simulink model "simRouteA_v4_11"  (R2015a)
settings: Solver=FixedStepDiscrete  StartTime=0.0  StopTime=36000  FixedStep=1  RelTol=1e-3
PreLoadFcn:
  | loadTimetable
StopFcn:
  | postProcess
undefined symbols (not defined in the file or in its folder): setBus1IntergenTime, setBus2IntergenTime, setBus3IntergenTime, setBus4IntergenTime
(part 3 of 7)

== system simRouteA_v4_11/inTransitLinkL10 ==
  xtraDelay : Inport
  theoTravTime : Inport  Port=2
  Add : Sum
  Buses being hold on the street : InfiniteServer  ServiceTimeFrom=Signal port t
  Clock2 : Clock
  DummyServer : SingleServer  ServiceTime=0
  FIFO Queue1 : FIFOQueue
  FIFO Queue3 : FIFOQueue
  FIFO Queue9 : FIFOQueue
  Get Attribute : GetAttribute  AttributeName=ID  EvaluatedDefaultAttributeValue={ []}
      settings: OutputPortMap=o1
  Get Attribute5 : GetAttribute  AttributeName=tTrav|time  AttributeMissing=Error|Error  AttributeDefaultValue=1|1  AttributeTreatAsVector=1|1  AttributeSendTiming=After entity departure|After entity departure  EvaluatedDefaultAttributeValue={ []; []}
      settings: OutputPortMap=o1,o2
  Set Attribute3 : SetAttribute  AttributeName=tTrav|time  AttributeFrom=Signal port|Signal port  AttributeValue=1|1  AttributeTreatAsVector=1|1  EvaluatedAttributeValue={ []; [] }
      settings: InputPortMap=u0,u1
  Subsystem2 : Subsystem  TreatAsAtomicUnit=on
  T2E4 : TimedToEventSignal
  busesOutLink : PMIOPort  Port=1  Side=Right
  busesHitTheRoad : PMIOPort  Port=2  Side=Left
  idBusOutLink : Outport
  wires:
  xtraDelay/1 -> Add/1
  theoTravTime/1 -> Add/2
  Add/1 -> Set Attribute3/1
  Get Attribute/1 -> idBusOutLink/1
  Clock2/1 -> T2E4/1
  T2E4/1 -> Set Attribute3/2
  Get Attribute5/1 -> Subsystem2/1(tTrav)
  Get Attribute5/2 -> Subsystem2/2(tDep)
  Subsystem2/1(tTravNew) -> Buses being hold on the street/1
  connections:
  Buses being hold on the street/RConn1 -- FIFO Queue9/LConn1
  FIFO Queue1/LConn1 -- busesHitTheRoad/RConn1
  Get Attribute/RConn1 -- busesOutLink/RConn1
  FIFO Queue9/RConn1 -- Get Attribute/LConn1
  FIFO Queue1/RConn1 -- Set Attribute3/LConn1
  Set Attribute3/RConn1 -- FIFO Queue3/LConn1
  FIFO Queue3/RConn1 -- Get Attribute5/LConn1
  Get Attribute5/RConn1 -- DummyServer/LConn1
  DummyServer/RConn1 -- Buses being hold on the street/LConn1

== system simRouteA_v4_11/inTransitLinkL11 ==
  xtraDelay : Inport
  theoTravTime : Inport  Port=2
  Add : Sum
  Buses being hold on the street : InfiniteServer  ServiceTimeFrom=Signal port t
  Clock2 : Clock
  DummyServer : SingleServer  ServiceTime=0
  FIFO Queue1 : FIFOQueue
  FIFO Queue3 : FIFOQueue
  FIFO Queue9 : FIFOQueue
  Get Attribute : GetAttribute  AttributeName=ID  EvaluatedDefaultAttributeValue={ []}
      settings: OutputPortMap=o1
  Get Attribute5 : GetAttribute  AttributeName=tTrav|time  AttributeMissing=Error|Error  AttributeDefaultValue=1|1  AttributeTreatAsVector=1|1  AttributeSendTiming=After entity departure|After entity departure  EvaluatedDefaultAttributeValue={ []; []}
      settings: OutputPortMap=o1,o2
  Set Attribute3 : SetAttribute  AttributeName=tTrav|time  AttributeFrom=Signal port|Signal port  AttributeValue=1|1  AttributeTreatAsVector=1|1  EvaluatedAttributeValue={ []; [] }
      settings: InputPortMap=u0,u1
  Subsystem2 : Subsystem  TreatAsAtomicUnit=on
  T2E4 : TimedToEventSignal
  busesOutLink : PMIOPort  Port=1  Side=Right
  busesHitTheRoad : PMIOPort  Port=2  Side=Left
  idBusOutLink : Outport
  wires:
  xtraDelay/1 -> Add/1
  theoTravTime/1 -> Add/2
  Add/1 -> Set Attribute3/1
  Get Attribute/1 -> idBusOutLink/1
  Clock2/1 -> T2E4/1
  T2E4/1 -> Set Attribute3/2
  Get Attribute5/1 -> Subsystem2/1(tTrav)
  Get Attribute5/2 -> Subsystem2/2(tDep)
  Subsystem2/1(tTravNew) -> Buses being hold on the street/1
  connections:
  Buses being hold on the street/RConn1 -- FIFO Queue9/LConn1
  FIFO Queue1/LConn1 -- busesHitTheRoad/RConn1
  Get Attribute/RConn1 -- busesOutLink/RConn1
  FIFO Queue9/RConn1 -- Get Attribute/LConn1
  FIFO Queue1/RConn1 -- Set Attribute3/LConn1
  Set Attribute3/RConn1 -- FIFO Queue3/LConn1
  FIFO Queue3/RConn1 -- Get Attribute5/LConn1
  Get Attribute5/RConn1 -- DummyServer/LConn1
  DummyServer/RConn1 -- Buses being hold on the street/LConn1

== system simRouteA_v4_11/inTransitLinkL12 ==
  xtraDelay : Inport
  theoTravTime : Inport  Port=2
  Add : Sum
  Buses being hold on the street : InfiniteServer  ServiceTimeFrom=Signal port t
  Clock2 : Clock
  DummyServer : SingleServer  ServiceTime=0
  FIFO Queue1 : FIFOQueue
  FIFO Queue3 : FIFOQueue
  FIFO Queue9 : FIFOQueue
  Get Attribute : GetAttribute  AttributeName=ID  EvaluatedDefaultAttributeValue={ []}
      settings: OutputPortMap=o1
  Get Attribute5 : GetAttribute  AttributeName=tTrav|time  AttributeMissing=Error|Error  AttributeDefaultValue=1|1  AttributeTreatAsVector=1|1  AttributeSendTiming=After entity departure|After entity departure  EvaluatedDefaultAttributeValue={ []; []}
      settings: OutputPortMap=o1,o2
  Set Attribute3 : SetAttribute  AttributeName=tTrav|time  AttributeFrom=Signal port|Signal port  AttributeValue=1|1  AttributeTreatAsVector=1|1  EvaluatedAttributeValue={ []; [] }
      settings: InputPortMap=u0,u1
  Subsystem2 : Subsystem  TreatAsAtomicUnit=on
  T2E4 : TimedToEventSignal
  busesOutLink : PMIOPort  Port=1  Side=Right
  busesHitTheRoad : PMIOPort  Port=2  Side=Left
  idBusOutLink : Outport
  wires:
  xtraDelay/1 -> Add/1
  theoTravTime/1 -> Add/2
  Add/1 -> Set Attribute3/1
  Get Attribute/1 -> idBusOutLink/1
  Clock2/1 -> T2E4/1
  T2E4/1 -> Set Attribute3/2
  Get Attribute5/1 -> Subsystem2/1(tTrav)
  Get Attribute5/2 -> Subsystem2/2(tDep)
  Subsystem2/1(tTravNew) -> Buses being hold on the street/1
  connections:
  Buses being hold on the street/RConn1 -- FIFO Queue9/LConn1
  FIFO Queue1/LConn1 -- busesHitTheRoad/RConn1
  Get Attribute/RConn1 -- busesOutLink/RConn1
  FIFO Queue9/RConn1 -- Get Attribute/LConn1
  FIFO Queue1/RConn1 -- Set Attribute3/LConn1
  Set Attribute3/RConn1 -- FIFO Queue3/LConn1
  FIFO Queue3/RConn1 -- Get Attribute5/LConn1
  Get Attribute5/RConn1 -- DummyServer/LConn1
  DummyServer/RConn1 -- Buses being hold on the street/LConn1

== system simRouteA_v4_11/inTransitLinkL13 ==
  xtraDelay : Inport
  theoTravTime : Inport  Port=2
  Add : Sum
  Buses being hold on the street : InfiniteServer  ServiceTimeFrom=Signal port t
  Clock2 : Clock
  DummyServer : SingleServer  ServiceTime=0
  FIFO Queue1 : FIFOQueue
  FIFO Queue3 : FIFOQueue
  FIFO Queue9 : FIFOQueue
  Get Attribute : GetAttribute  AttributeName=ID  EvaluatedDefaultAttributeValue={ []}
      settings: OutputPortMap=o1
  Get Attribute5 : GetAttribute  AttributeName=tTrav|time  AttributeMissing=Error|Error  AttributeDefaultValue=1|1  AttributeTreatAsVector=1|1  AttributeSendTiming=After entity departure|After entity departure  EvaluatedDefaultAttributeValue={ []; []}
      settings: OutputPortMap=o1,o2
  Set Attribute3 : SetAttribute  AttributeName=tTrav|time  AttributeFrom=Signal port|Signal port  AttributeValue=1|1  AttributeTreatAsVector=1|1  EvaluatedAttributeValue={ []; [] }
      settings: InputPortMap=u0,u1
  Subsystem2 : Subsystem  TreatAsAtomicUnit=on
  T2E4 : TimedToEventSignal
  busesOutLink : PMIOPort  Port=1  Side=Right
  busesHitTheRoad : PMIOPort  Port=2  Side=Left
  idBusOutLink : Outport
  wires:
  xtraDelay/1 -> Add/1
  theoTravTime/1 -> Add/2
  Add/1 -> Set Attribute3/1
  Get Attribute/1 -> idBusOutLink/1
  Clock2/1 -> T2E4/1
  T2E4/1 -> Set Attribute3/2
  Get Attribute5/1 -> Subsystem2/1(tTrav)
  Get Attribute5/2 -> Subsystem2/2(tDep)
  Subsystem2/1(tTravNew) -> Buses being hold on the street/1
  connections:
  Buses being hold on the street/RConn1 -- FIFO Queue9/LConn1
  FIFO Queue1/LConn1 -- busesHitTheRoad/RConn1
  Get Attribute/RConn1 -- busesOutLink/RConn1
  FIFO Queue9/RConn1 -- Get Attribute/LConn1
  FIFO Queue1/RConn1 -- Set Attribute3/LConn1
  Set Attribute3/RConn1 -- FIFO Queue3/LConn1
  FIFO Queue3/RConn1 -- Get Attribute5/LConn1
  Get Attribute5/RConn1 -- DummyServer/LConn1
  DummyServer/RConn1 -- Buses being hold on the street/LConn1

== system simRouteA_v4_11/inTransitLinkL14 ==
  xtraDelay : Inport
  theoTravTime : Inport  Port=2
  Add : Sum
  Buses being hold on the street : InfiniteServer  ServiceTimeFrom=Signal port t
  Clock2 : Clock
  DummyServer : SingleServer  ServiceTime=0
  FIFO Queue1 : FIFOQueue
  FIFO Queue3 : FIFOQueue
  FIFO Queue9 : FIFOQueue
  Get Attribute : GetAttribute  AttributeName=ID  EvaluatedDefaultAttributeValue={ []}
      settings: OutputPortMap=o1
  Get Attribute5 : GetAttribute  AttributeName=tTrav|time  AttributeMissing=Error|Error  AttributeDefaultValue=1|1  AttributeTreatAsVector=1|1  AttributeSendTiming=After entity departure|After entity departure  EvaluatedDefaultAttributeValue={ []; []}
      settings: OutputPortMap=o1,o2
  Set Attribute3 : SetAttribute  AttributeName=tTrav|time  AttributeFrom=Signal port|Signal port  AttributeValue=1|1  AttributeTreatAsVector=1|1  EvaluatedAttributeValue={ []; [] }
      settings: InputPortMap=u0,u1
  Subsystem2 : Subsystem  TreatAsAtomicUnit=on
  T2E4 : TimedToEventSignal
  busesOutLink : PMIOPort  Port=1  Side=Right
  busesHitTheRoad : PMIOPort  Port=2  Side=Left
  idBusOutLink : Outport
  wires:
  xtraDelay/1 -> Add/1
  theoTravTime/1 -> Add/2
  Add/1 -> Set Attribute3/1
  Get Attribute/1 -> idBusOutLink/1
  Clock2/1 -> T2E4/1
  T2E4/1 -> Set Attribute3/2
  Get Attribute5/1 -> Subsystem2/1(tTrav)
  Get Attribute5/2 -> Subsystem2/2(tDep)
  Subsystem2/1(tTravNew) -> Buses being hold on the street/1
  connections:
  Buses being hold on the street/RConn1 -- FIFO Queue9/LConn1
  FIFO Queue1/LConn1 -- busesHitTheRoad/RConn1
  Get Attribute/RConn1 -- busesOutLink/RConn1
  FIFO Queue9/RConn1 -- Get Attribute/LConn1
  FIFO Queue1/RConn1 -- Set Attribute3/LConn1
  Set Attribute3/RConn1 -- FIFO Queue3/LConn1
  FIFO Queue3/RConn1 -- Get Attribute5/LConn1
  Get Attribute5/RConn1 -- DummyServer/LConn1
  DummyServer/RConn1 -- Buses being hold on the street/LConn1

== system simRouteA_v4_11/inTransitLinkL15 ==
  xtraDelay : Inport
  theoTravTime : Inport  Port=2
  Add : Sum
  Buses being hold on the street : InfiniteServer  ServiceTimeFrom=Signal port t
  Clock2 : Clock
  DummyServer : SingleServer  ServiceTime=0
  FIFO Queue1 : FIFOQueue
  FIFO Queue3 : FIFOQueue
  FIFO Queue9 : FIFOQueue
  Get Attribute : GetAttribute  AttributeName=ID  EvaluatedDefaultAttributeValue={ []}
      settings: OutputPortMap=o1
  Get Attribute5 : GetAttribute  AttributeName=tTrav|time  AttributeMissing=Error|Error  AttributeDefaultValue=1|1  AttributeTreatAsVector=1|1  AttributeSendTiming=After entity departure|After entity departure  EvaluatedDefaultAttributeValue={ []; []}
      settings: OutputPortMap=o1,o2
  Set Attribute3 : SetAttribute  AttributeName=tTrav|time  AttributeFrom=Signal port|Signal port  AttributeValue=1|1  AttributeTreatAsVector=1|1  EvaluatedAttributeValue={ []; [] }
      settings: InputPortMap=u0,u1
  Subsystem2 : Subsystem  TreatAsAtomicUnit=on
  T2E4 : TimedToEventSignal
  busesOutLink : PMIOPort  Port=1  Side=Right
  busesHitTheRoad : PMIOPort  Port=2  Side=Left
  idBusOutLink : Outport
  wires:
  xtraDelay/1 -> Add/1
  theoTravTime/1 -> Add/2
  Add/1 -> Set Attribute3/1
  Get Attribute/1 -> idBusOutLink/1
  Clock2/1 -> T2E4/1
  T2E4/1 -> Set Attribute3/2
  Get Attribute5/1 -> Subsystem2/1(tTrav)
  Get Attribute5/2 -> Subsystem2/2(tDep)
  Subsystem2/1(tTravNew) -> Buses being hold on the street/1
  connections:
  Buses being hold on the street/RConn1 -- FIFO Queue9/LConn1
  FIFO Queue1/LConn1 -- busesHitTheRoad/RConn1
  Get Attribute/RConn1 -- busesOutLink/RConn1
  FIFO Queue9/RConn1 -- Get Attribute/LConn1
  FIFO Queue1/RConn1 -- Set Attribute3/LConn1
  Set Attribute3/RConn1 -- FIFO Queue3/LConn1
  FIFO Queue3/RConn1 -- Get Attribute5/LConn1
  Get Attribute5/RConn1 -- DummyServer/LConn1
  DummyServer/RConn1 -- Buses being hold on the street/LConn1

== system simRouteA_v4_11/inTransitLinkL16 ==
  xtraDelay : Inport
  theoTravTime : Inport  Port=2
  Add : Sum
  Buses being hold on the street : InfiniteServer  ServiceTimeFrom=Signal port t
  Clock2 : Clock
  DummyServer : SingleServer  ServiceTime=0
  FIFO Queue1 : FIFOQueue
  FIFO Queue3 : FIFOQueue
  FIFO Queue9 : FIFOQueue
  Get Attribute : GetAttribute  AttributeName=ID  EvaluatedDefaultAttributeValue={ []}
      settings: OutputPortMap=o1
  Get Attribute5 : GetAttribute  AttributeName=tTrav|time  AttributeMissing=Error|Error  AttributeDefaultValue=1|1  AttributeTreatAsVector=1|1  AttributeSendTiming=After entity departure|After entity departure  EvaluatedDefaultAttributeValue={ []; []}
      settings: OutputPortMap=o1,o2
  Set Attribute3 : SetAttribute  AttributeName=tTrav|time  AttributeFrom=Signal port|Signal port  AttributeValue=1|1  AttributeTreatAsVector=1|1  EvaluatedAttributeValue={ []; [] }
      settings: InputPortMap=u0,u1
  Subsystem2 : Subsystem  TreatAsAtomicUnit=on
  T2E4 : TimedToEventSignal
  busesOutLink : PMIOPort  Port=1  Side=Right
  busesHitTheRoad : PMIOPort  Port=2  Side=Left
  idBusOutLink : Outport
  wires:
  xtraDelay/1 -> Add/1
  theoTravTime/1 -> Add/2
  Add/1 -> Set Attribute3/1
  Get Attribute/1 -> idBusOutLink/1
  Clock2/1 -> T2E4/1
  T2E4/1 -> Set Attribute3/2
  Get Attribute5/1 -> Subsystem2/1(tTrav)
  Get Attribute5/2 -> Subsystem2/2(tDep)
  Subsystem2/1(tTravNew) -> Buses being hold on the street/1
  connections:
  Buses being hold on the street/RConn1 -- FIFO Queue9/LConn1
  FIFO Queue1/LConn1 -- busesHitTheRoad/RConn1
  Get Attribute/RConn1 -- busesOutLink/RConn1
  FIFO Queue9/RConn1 -- Get Attribute/LConn1
  FIFO Queue1/RConn1 -- Set Attribute3/LConn1
  Set Attribute3/RConn1 -- FIFO Queue3/LConn1
  FIFO Queue3/RConn1 -- Get Attribute5/LConn1
  Get Attribute5/RConn1 -- DummyServer/LConn1
  DummyServer/RConn1 -- Buses being hold on the street/LConn1

== system simRouteA_v4_11/inTransitLinkL17 ==
  xtraDelay : Inport
  theoTravTime : Inport  Port=2
  Add : Sum
  Buses being hold on the street : InfiniteServer  ServiceTimeFrom=Signal port t
  Clock2 : Clock
  DummyServer : SingleServer  ServiceTime=0
  FIFO Queue1 : FIFOQueue
  FIFO Queue3 : FIFOQueue
  FIFO Queue9 : FIFOQueue
  Get Attribute : GetAttribute  AttributeName=ID  EvaluatedDefaultAttributeValue={ []}
      settings: OutputPortMap=o1
  Get Attribute5 : GetAttribute  AttributeName=tTrav|time  AttributeMissing=Error|Error  AttributeDefaultValue=1|1  AttributeTreatAsVector=1|1  AttributeSendTiming=After entity departure|After entity departure  EvaluatedDefaultAttributeValue={ []; []}
      settings: OutputPortMap=o1,o2
  Set Attribute3 : SetAttribute  AttributeName=tTrav|time  AttributeFrom=Signal port|Signal port  AttributeValue=1|1  AttributeTreatAsVector=1|1  EvaluatedAttributeValue={ []; [] }
      settings: InputPortMap=u0,u1
  Subsystem2 : Subsystem  TreatAsAtomicUnit=on
  T2E4 : TimedToEventSignal
  busesOutLink : PMIOPort  Port=1  Side=Right
  busesHitTheRoad : PMIOPort  Port=2  Side=Left
  idBusOutLink : Outport
  wires:
  xtraDelay/1 -> Add/1
  theoTravTime/1 -> Add/2
  Add/1 -> Set Attribute3/1
  Get Attribute/1 -> idBusOutLink/1
  Clock2/1 -> T2E4/1
  T2E4/1 -> Set Attribute3/2
  Get Attribute5/1 -> Subsystem2/1(tTrav)
  Get Attribute5/2 -> Subsystem2/2(tDep)
  Subsystem2/1(tTravNew) -> Buses being hold on the street/1
  connections:
  Buses being hold on the street/RConn1 -- FIFO Queue9/LConn1
  FIFO Queue1/LConn1 -- busesHitTheRoad/RConn1
  Get Attribute/RConn1 -- busesOutLink/RConn1
  FIFO Queue9/RConn1 -- Get Attribute/LConn1
  FIFO Queue1/RConn1 -- Set Attribute3/LConn1
  Set Attribute3/RConn1 -- FIFO Queue3/LConn1
  FIFO Queue3/RConn1 -- Get Attribute5/LConn1
  Get Attribute5/RConn1 -- DummyServer/LConn1
  DummyServer/RConn1 -- Buses being hold on the street/LConn1

== system simRouteA_v4_11/inTransitLinkL18 ==
  xtraDelay : Inport
  theoTravTime : Inport  Port=2
  Add : Sum
  Buses being hold on the street : InfiniteServer  ServiceTimeFrom=Signal port t
  Clock2 : Clock
  DummyServer : SingleServer  ServiceTime=0
  FIFO Queue1 : FIFOQueue
  FIFO Queue3 : FIFOQueue
  FIFO Queue9 : FIFOQueue
  Get Attribute : GetAttribute  AttributeName=ID  EvaluatedDefaultAttributeValue={ []}
      settings: OutputPortMap=o1
  Get Attribute5 : GetAttribute  AttributeName=tTrav|time  AttributeMissing=Error|Error  AttributeDefaultValue=1|1  AttributeTreatAsVector=1|1  AttributeSendTiming=After entity departure|After entity departure  EvaluatedDefaultAttributeValue={ []; []}
      settings: OutputPortMap=o1,o2
  Set Attribute3 : SetAttribute  AttributeName=tTrav|time  AttributeFrom=Signal port|Signal port  AttributeValue=1|1  AttributeTreatAsVector=1|1  EvaluatedAttributeValue={ []; [] }
      settings: InputPortMap=u0,u1
  Subsystem2 : Subsystem  TreatAsAtomicUnit=on
  T2E4 : TimedToEventSignal
  busesOutLink : PMIOPort  Port=1  Side=Right
  busesHitTheRoad : PMIOPort  Port=2  Side=Left
  idBusOutLink : Outport
  wires:
  xtraDelay/1 -> Add/1
  theoTravTime/1 -> Add/2
  Add/1 -> Set Attribute3/1
  Get Attribute/1 -> idBusOutLink/1
  Clock2/1 -> T2E4/1
  T2E4/1 -> Set Attribute3/2
  Get Attribute5/1 -> Subsystem2/1(tTrav)
  Get Attribute5/2 -> Subsystem2/2(tDep)
  Subsystem2/1(tTravNew) -> Buses being hold on the street/1
  connections:
  Buses being hold on the street/RConn1 -- FIFO Queue9/LConn1
  FIFO Queue1/LConn1 -- busesHitTheRoad/RConn1
  Get Attribute/RConn1 -- busesOutLink/RConn1
  FIFO Queue9/RConn1 -- Get Attribute/LConn1
  FIFO Queue1/RConn1 -- Set Attribute3/LConn1
  Set Attribute3/RConn1 -- FIFO Queue3/LConn1
  FIFO Queue3/RConn1 -- Get Attribute5/LConn1
  Get Attribute5/RConn1 -- DummyServer/LConn1
  DummyServer/RConn1 -- Buses being hold on the street/LConn1

== system simRouteA_v4_11/inTransitLinkL2 ==
  xtraDelay : Inport
  theoTravTime : Inport  Port=2
  Add : Sum
  Buses being hold on the street : InfiniteServer  ServiceTimeFrom=Signal port t
  Clock2 : Clock
  DummyServer : SingleServer  ServiceTime=0
  FIFO Queue1 : FIFOQueue
  FIFO Queue3 : FIFOQueue
  FIFO Queue9 : FIFOQueue
  Get Attribute : GetAttribute  AttributeName=ID  EvaluatedDefaultAttributeValue={ []}
      settings: OutputPortMap=o1
  Get Attribute5 : GetAttribute  AttributeName=tTrav|time  AttributeMissing=Error|Error  AttributeDefaultValue=1|1  AttributeTreatAsVector=1|1  AttributeSendTiming=After entity departure|After entity departure  EvaluatedDefaultAttributeValue={ []; []}
      settings: OutputPortMap=o1,o2
  Set Attribute3 : SetAttribute  AttributeName=tTrav|time  AttributeFrom=Signal port|Signal port  AttributeValue=1|1  AttributeTreatAsVector=1|1  EvaluatedAttributeValue={ []; [] }
      settings: InputPortMap=u0,u1
  Subsystem2 : Subsystem  TreatAsAtomicUnit=on
  T2E4 : TimedToEventSignal
  busesOutLink : PMIOPort  Port=1  Side=Right
  busesHitTheRoad : PMIOPort  Port=2  Side=Left
  idBusOutLink : Outport
  wires:
  xtraDelay/1 -> Add/1
  theoTravTime/1 -> Add/2
  Add/1 -> Set Attribute3/1
  Get Attribute/1 -> idBusOutLink/1
  Clock2/1 -> T2E4/1
  T2E4/1 -> Set Attribute3/2
  Get Attribute5/1 -> Subsystem2/1(tTrav)
  Get Attribute5/2 -> Subsystem2/2(tDep)
  Subsystem2/1(tTravNew) -> Buses being hold on the street/1
  connections:
  Buses being hold on the street/RConn1 -- FIFO Queue9/LConn1
  FIFO Queue1/LConn1 -- busesHitTheRoad/RConn1
  Get Attribute/RConn1 -- busesOutLink/RConn1
  FIFO Queue9/RConn1 -- Get Attribute/LConn1
  FIFO Queue1/RConn1 -- Set Attribute3/LConn1
  Set Attribute3/RConn1 -- FIFO Queue3/LConn1
  FIFO Queue3/RConn1 -- Get Attribute5/LConn1
  Get Attribute5/RConn1 -- DummyServer/LConn1
  DummyServer/RConn1 -- Buses being hold on the street/LConn1

== system simRouteA_v4_11/inTransitLinkL3 ==
  xtraDelay : Inport
  theoTravTime : Inport  Port=2
  Add : Sum
  Buses being hold on the street : InfiniteServer  ServiceTimeFrom=Signal port t
  Clock2 : Clock
  DummyServer : SingleServer  ServiceTime=0
  FIFO Queue1 : FIFOQueue
  FIFO Queue3 : FIFOQueue
  FIFO Queue9 : FIFOQueue
  Get Attribute : GetAttribute  AttributeName=ID  EvaluatedDefaultAttributeValue={ []}
      settings: OutputPortMap=o1
  Get Attribute5 : GetAttribute  AttributeName=tTrav|time  AttributeMissing=Error|Error  AttributeDefaultValue=1|1  AttributeTreatAsVector=1|1  AttributeSendTiming=After entity departure|After entity departure  EvaluatedDefaultAttributeValue={ []; []}
      settings: OutputPortMap=o1,o2
  Set Attribute3 : SetAttribute  AttributeName=tTrav|time  AttributeFrom=Signal port|Signal port  AttributeValue=1|1  AttributeTreatAsVector=1|1  EvaluatedAttributeValue={ []; [] }
      settings: InputPortMap=u0,u1
  Subsystem2 : Subsystem  TreatAsAtomicUnit=on
  T2E4 : TimedToEventSignal
  busesOutLink : PMIOPort  Port=1  Side=Right
  busesHitTheRoad : PMIOPort  Port=2  Side=Left
  idBusOutLink : Outport
  wires:
  xtraDelay/1 -> Add/1
  theoTravTime/1 -> Add/2
  Add/1 -> Set Attribute3/1
  Get Attribute/1 -> idBusOutLink/1
  Clock2/1 -> T2E4/1
  T2E4/1 -> Set Attribute3/2
  Get Attribute5/1 -> Subsystem2/1(tTrav)
  Get Attribute5/2 -> Subsystem2/2(tDep)
  Subsystem2/1(tTravNew) -> Buses being hold on the street/1
  connections:
  Buses being hold on the street/RConn1 -- FIFO Queue9/LConn1
  FIFO Queue1/LConn1 -- busesHitTheRoad/RConn1
  Get Attribute/RConn1 -- busesOutLink/RConn1
  FIFO Queue9/RConn1 -- Get Attribute/LConn1
  FIFO Queue1/RConn1 -- Set Attribute3/LConn1
  Set Attribute3/RConn1 -- FIFO Queue3/LConn1
  FIFO Queue3/RConn1 -- Get Attribute5/LConn1
  Get Attribute5/RConn1 -- DummyServer/LConn1
  DummyServer/RConn1 -- Buses being hold on the street/LConn1

== system simRouteA_v4_11/inTransitLinkL4 ==
  xtraDelay : Inport
  theoTravTime : Inport  Port=2
  Add : Sum
  Buses being hold on the street : InfiniteServer  ServiceTimeFrom=Signal port t
  Clock2 : Clock
  DummyServer : SingleServer  ServiceTime=0
  FIFO Queue1 : FIFOQueue
  FIFO Queue3 : FIFOQueue
  FIFO Queue9 : FIFOQueue
  Get Attribute : GetAttribute  AttributeName=ID  EvaluatedDefaultAttributeValue={ []}
      settings: OutputPortMap=o1
  Get Attribute5 : GetAttribute  AttributeName=tTrav|time  AttributeMissing=Error|Error  AttributeDefaultValue=1|1  AttributeTreatAsVector=1|1  AttributeSendTiming=After entity departure|After entity departure  EvaluatedDefaultAttributeValue={ []; []}
      settings: OutputPortMap=o1,o2
  Set Attribute3 : SetAttribute  AttributeName=tTrav|time  AttributeFrom=Signal port|Signal port  AttributeValue=1|1  AttributeTreatAsVector=1|1  EvaluatedAttributeValue={ []; [] }
      settings: InputPortMap=u0,u1
  Subsystem2 : Subsystem  TreatAsAtomicUnit=on
  T2E4 : TimedToEventSignal
  busesOutLink : PMIOPort  Port=1  Side=Right
  busesHitTheRoad : PMIOPort  Port=2  Side=Left
  idBusOutLink : Outport
  wires:
  xtraDelay/1 -> Add/1
  theoTravTime/1 -> Add/2
  Add/1 -> Set Attribute3/1
  Get Attribute/1 -> idBusOutLink/1
  Clock2/1 -> T2E4/1
  T2E4/1 -> Set Attribute3/2
  Get Attribute5/1 -> Subsystem2/1(tTrav)
  Get Attribute5/2 -> Subsystem2/2(tDep)
  Subsystem2/1(tTravNew) -> Buses being hold on the street/1
  connections:
  Buses being hold on the street/RConn1 -- FIFO Queue9/LConn1
  FIFO Queue1/LConn1 -- busesHitTheRoad/RConn1
  Get Attribute/RConn1 -- busesOutLink/RConn1
  FIFO Queue9/RConn1 -- Get Attribute/LConn1
  FIFO Queue1/RConn1 -- Set Attribute3/LConn1
  Set Attribute3/RConn1 -- FIFO Queue3/LConn1
  FIFO Queue3/RConn1 -- Get Attribute5/LConn1
  Get Attribute5/RConn1 -- DummyServer/LConn1
  DummyServer/RConn1 -- Buses being hold on the street/LConn1

== system simRouteA_v4_11/inTransitLinkL5 ==
  xtraDelay : Inport
  theoTravTime : Inport  Port=2
  Add : Sum
  Buses being hold on the street : InfiniteServer  ServiceTimeFrom=Signal port t
  Clock2 : Clock
  DummyServer : SingleServer  ServiceTime=0
  FIFO Queue1 : FIFOQueue
  FIFO Queue3 : FIFOQueue
  FIFO Queue9 : FIFOQueue
  Get Attribute : GetAttribute  AttributeName=ID  EvaluatedDefaultAttributeValue={ []}
      settings: OutputPortMap=o1
  Get Attribute5 : GetAttribute  AttributeName=tTrav|time  AttributeMissing=Error|Error  AttributeDefaultValue=1|1  AttributeTreatAsVector=1|1  AttributeSendTiming=After entity departure|After entity departure  EvaluatedDefaultAttributeValue={ []; []}
      settings: OutputPortMap=o1,o2
  Set Attribute3 : SetAttribute  AttributeName=tTrav|time  AttributeFrom=Signal port|Signal port  AttributeValue=1|1  AttributeTreatAsVector=1|1  EvaluatedAttributeValue={ []; [] }
      settings: InputPortMap=u0,u1
  Subsystem2 : Subsystem  TreatAsAtomicUnit=on
  T2E4 : TimedToEventSignal
  busesOutLink : PMIOPort  Port=1  Side=Right
  busesHitTheRoad : PMIOPort  Port=2  Side=Left
  idBusOutLink : Outport
  wires:
  xtraDelay/1 -> Add/1
  theoTravTime/1 -> Add/2
  Add/1 -> Set Attribute3/1
  Get Attribute/1 -> idBusOutLink/1
  Clock2/1 -> T2E4/1
  T2E4/1 -> Set Attribute3/2
  Get Attribute5/1 -> Subsystem2/1(tTrav)
  Get Attribute5/2 -> Subsystem2/2(tDep)
  Subsystem2/1(tTravNew) -> Buses being hold on the street/1
  connections:
  Buses being hold on the street/RConn1 -- FIFO Queue9/LConn1
  FIFO Queue1/LConn1 -- busesHitTheRoad/RConn1
  Get Attribute/RConn1 -- busesOutLink/RConn1
  FIFO Queue9/RConn1 -- Get Attribute/LConn1
  FIFO Queue1/RConn1 -- Set Attribute3/LConn1
  Set Attribute3/RConn1 -- FIFO Queue3/LConn1
  FIFO Queue3/RConn1 -- Get Attribute5/LConn1
  Get Attribute5/RConn1 -- DummyServer/LConn1
  DummyServer/RConn1 -- Buses being hold on the street/LConn1

== system simRouteA_v4_11/inTransitLinkL6 ==
  xtraDelay : Inport
  theoTravTime : Inport  Port=2
  Add : Sum
  Buses being hold on the street : InfiniteServer  ServiceTimeFrom=Signal port t
  Clock2 : Clock
  DummyServer : SingleServer  ServiceTime=0
  FIFO Queue1 : FIFOQueue
  FIFO Queue3 : FIFOQueue
  FIFO Queue9 : FIFOQueue
  Get Attribute : GetAttribute  AttributeName=ID  EvaluatedDefaultAttributeValue={ []}
      settings: OutputPortMap=o1
  Get Attribute5 : GetAttribute  AttributeName=tTrav|time  AttributeMissing=Error|Error  AttributeDefaultValue=1|1  AttributeTreatAsVector=1|1  AttributeSendTiming=After entity departure|After entity departure  EvaluatedDefaultAttributeValue={ []; []}
      settings: OutputPortMap=o1,o2
  Set Attribute3 : SetAttribute  AttributeName=tTrav|time  AttributeFrom=Signal port|Signal port  AttributeValue=1|1  AttributeTreatAsVector=1|1  EvaluatedAttributeValue={ []; [] }
      settings: InputPortMap=u0,u1
  Subsystem2 : Subsystem  TreatAsAtomicUnit=on
  T2E4 : TimedToEventSignal
  busesOutLink : PMIOPort  Port=1  Side=Right
  busesHitTheRoad : PMIOPort  Port=2  Side=Left
  idBusOutLink : Outport
  wires:
  xtraDelay/1 -> Add/1
  theoTravTime/1 -> Add/2
  Add/1 -> Set Attribute3/1
  Get Attribute/1 -> idBusOutLink/1
  Clock2/1 -> T2E4/1
  T2E4/1 -> Set Attribute3/2
  Get Attribute5/1 -> Subsystem2/1(tTrav)
  Get Attribute5/2 -> Subsystem2/2(tDep)
  Subsystem2/1(tTravNew) -> Buses being hold on the street/1
  connections:
  Buses being hold on the street/RConn1 -- FIFO Queue9/LConn1
  FIFO Queue1/LConn1 -- busesHitTheRoad/RConn1
  Get Attribute/RConn1 -- busesOutLink/RConn1
  FIFO Queue9/RConn1 -- Get Attribute/LConn1
  FIFO Queue1/RConn1 -- Set Attribute3/LConn1
  Set Attribute3/RConn1 -- FIFO Queue3/LConn1
  FIFO Queue3/RConn1 -- Get Attribute5/LConn1
  Get Attribute5/RConn1 -- DummyServer/LConn1
  DummyServer/RConn1 -- Buses being hold on the street/LConn1

== system simRouteA_v4_11/inTransitLinkL7 ==
  xtraDelay : Inport
  theoTravTime : Inport  Port=2
  Add : Sum
  Buses being hold on the street : InfiniteServer  ServiceTimeFrom=Signal port t
  Clock2 : Clock
  DummyServer : SingleServer  ServiceTime=0
  FIFO Queue1 : FIFOQueue
  FIFO Queue3 : FIFOQueue
  FIFO Queue9 : FIFOQueue
  Get Attribute : GetAttribute  AttributeName=ID  EvaluatedDefaultAttributeValue={ []}
      settings: OutputPortMap=o1
  Get Attribute5 : GetAttribute  AttributeName=tTrav|time  AttributeMissing=Error|Error  AttributeDefaultValue=1|1  AttributeTreatAsVector=1|1  AttributeSendTiming=After entity departure|After entity departure  EvaluatedDefaultAttributeValue={ []; []}
      settings: OutputPortMap=o1,o2
  Set Attribute3 : SetAttribute  AttributeName=tTrav|time  AttributeFrom=Signal port|Signal port  AttributeValue=1|1  AttributeTreatAsVector=1|1  EvaluatedAttributeValue={ []; [] }
      settings: InputPortMap=u0,u1
  Subsystem2 : Subsystem  TreatAsAtomicUnit=on
  T2E4 : TimedToEventSignal
  busesOutLink : PMIOPort  Port=1  Side=Right
  busesHitTheRoad : PMIOPort  Port=2  Side=Left
  idBusOutLink : Outport
  wires:
  xtraDelay/1 -> Add/1
  theoTravTime/1 -> Add/2
  Add/1 -> Set Attribute3/1
  Get Attribute/1 -> idBusOutLink/1
  Clock2/1 -> T2E4/1
  T2E4/1 -> Set Attribute3/2
  Get Attribute5/1 -> Subsystem2/1(tTrav)
  Get Attribute5/2 -> Subsystem2/2(tDep)
  Subsystem2/1(tTravNew) -> Buses being hold on the street/1
  connections:
  Buses being hold on the street/RConn1 -- FIFO Queue9/LConn1
  FIFO Queue1/LConn1 -- busesHitTheRoad/RConn1
  Get Attribute/RConn1 -- busesOutLink/RConn1
  FIFO Queue9/RConn1 -- Get Attribute/LConn1
  FIFO Queue1/RConn1 -- Set Attribute3/LConn1
  Set Attribute3/RConn1 -- FIFO Queue3/LConn1
  FIFO Queue3/RConn1 -- Get Attribute5/LConn1
  Get Attribute5/RConn1 -- DummyServer/LConn1
  DummyServer/RConn1 -- Buses being hold on the street/LConn1

== system simRouteA_v4_11/inTransitLinkL8 ==
  xtraDelay : Inport
  theoTravTime : Inport  Port=2
  Add : Sum
  Buses being hold on the street : InfiniteServer  ServiceTimeFrom=Signal port t
  Clock2 : Clock
  DummyServer : SingleServer  ServiceTime=0
  FIFO Queue1 : FIFOQueue
  FIFO Queue3 : FIFOQueue
  FIFO Queue9 : FIFOQueue
  Get Attribute : GetAttribute  AttributeName=ID  EvaluatedDefaultAttributeValue={ []}
      settings: OutputPortMap=o1
  Get Attribute5 : GetAttribute  AttributeName=tTrav|time  AttributeMissing=Error|Error  AttributeDefaultValue=1|1  AttributeTreatAsVector=1|1  AttributeSendTiming=After entity departure|After entity departure  EvaluatedDefaultAttributeValue={ []; []}
      settings: OutputPortMap=o1,o2
  Set Attribute3 : SetAttribute  AttributeName=tTrav|time  AttributeFrom=Signal port|Signal port  AttributeValue=1|1  AttributeTreatAsVector=1|1  EvaluatedAttributeValue={ []; [] }
      settings: InputPortMap=u0,u1
  Subsystem2 : Subsystem  TreatAsAtomicUnit=on
  T2E4 : TimedToEventSignal
  busesOutLink : PMIOPort  Port=1  Side=Right
  busesHitTheRoad : PMIOPort  Port=2  Side=Left
  idBusOutLink : Outport
  wires:
  xtraDelay/1 -> Add/1
  theoTravTime/1 -> Add/2
  Add/1 -> Set Attribute3/1
  Get Attribute/1 -> idBusOutLink/1
  Clock2/1 -> T2E4/1
  T2E4/1 -> Set Attribute3/2
  Get Attribute5/1 -> Subsystem2/1(tTrav)
  Get Attribute5/2 -> Subsystem2/2(tDep)
  Subsystem2/1(tTravNew) -> Buses being hold on the street/1
  connections:
  Buses being hold on the street/RConn1 -- FIFO Queue9/LConn1
  FIFO Queue1/LConn1 -- busesHitTheRoad/RConn1
  Get Attribute/RConn1 -- busesOutLink/RConn1
  FIFO Queue9/RConn1 -- Get Attribute/LConn1
  FIFO Queue1/RConn1 -- Set Attribute3/LConn1
  Set Attribute3/RConn1 -- FIFO Queue3/LConn1
  FIFO Queue3/RConn1 -- Get Attribute5/LConn1
  Get Attribute5/RConn1 -- DummyServer/LConn1
  DummyServer/RConn1 -- Buses being hold on the street/LConn1

== system simRouteA_v4_11/inTransitLinkL9 ==
  xtraDelay : Inport
  theoTravTime : Inport  Port=2
  Add : Sum
  Buses being hold on the street : InfiniteServer  ServiceTimeFrom=Signal port t
  Clock2 : Clock
  DummyServer : SingleServer  ServiceTime=0
  FIFO Queue1 : FIFOQueue
  FIFO Queue3 : FIFOQueue
  FIFO Queue9 : FIFOQueue
  Get Attribute : GetAttribute  AttributeName=ID  EvaluatedDefaultAttributeValue={ []}
      settings: OutputPortMap=o1
  Get Attribute5 : GetAttribute  AttributeName=tTrav|time  AttributeMissing=Error|Error  AttributeDefaultValue=1|1  AttributeTreatAsVector=1|1  AttributeSendTiming=After entity departure|After entity departure  EvaluatedDefaultAttributeValue={ []; []}
      settings: OutputPortMap=o1,o2
  Set Attribute3 : SetAttribute  AttributeName=tTrav|time  AttributeFrom=Signal port|Signal port  AttributeValue=1|1  AttributeTreatAsVector=1|1  EvaluatedAttributeValue={ []; [] }
      settings: InputPortMap=u0,u1
  Subsystem2 : Subsystem  TreatAsAtomicUnit=on
  T2E4 : TimedToEventSignal
  busesOutLink : PMIOPort  Port=1  Side=Right
  busesHitTheRoad : PMIOPort  Port=2  Side=Left
  idBusOutLink : Outport
  wires:
  xtraDelay/1 -> Add/1
  theoTravTime/1 -> Add/2
  Add/1 -> Set Attribute3/1
  Get Attribute/1 -> idBusOutLink/1
  Clock2/1 -> T2E4/1
  T2E4/1 -> Set Attribute3/2
  Get Attribute5/1 -> Subsystem2/1(tTrav)
  Get Attribute5/2 -> Subsystem2/2(tDep)
  Subsystem2/1(tTravNew) -> Buses being hold on the street/1
  connections:
  Buses being hold on the street/RConn1 -- FIFO Queue9/LConn1
  FIFO Queue1/LConn1 -- busesHitTheRoad/RConn1
  Get Attribute/RConn1 -- busesOutLink/RConn1
  FIFO Queue9/RConn1 -- Get Attribute/LConn1
  FIFO Queue1/RConn1 -- Set Attribute3/LConn1
  Set Attribute3/RConn1 -- FIFO Queue3/LConn1
  FIFO Queue3/RConn1 -- Get Attribute5/LConn1
  Get Attribute5/RConn1 -- DummyServer/LConn1
  DummyServer/RConn1 -- Buses being hold on the street/LConn1

== system simRouteA_v4_11/atStopS1/busDwellThisStop ==
  dwellTime : Inport
  Clock2 : Clock
  DummyServer : SingleServer  ServiceTime=0
  FIFO Queue3 : FIFOQueue
  Get Attribute5 : GetAttribute  AttributeName=dwellTime|tStartSrvPax  AttributeMissing=Error|Error  AttributeDefaultValue=1|1  AttributeTreatAsVector=1|1  AttributeSendTiming=After entity departure|After entity departure  EvaluatedDefaultAttributeValue={ []; []}
      settings: OutputPortMap=o1,o2
  Infinite Server : InfiniteServer  ServiceTimeFrom=Signal port t
  Set Attribute3 : SetAttribute  AttributeName=dwellTime|tStartSrvPax  AttributeFrom=Signal port|Signal port  AttributeValue=1|1  AttributeTreatAsVector=1|1  EvaluatedAttributeValue={ []; [] }
      settings: InputPortMap=u0,u1
  Subsystem2 : Subsystem  TreatAsAtomicUnit=on
  T2E4 : TimedToEventSignal
  busWaitAtStop : SingleServer  Commented=on  ServiceTimeFrom=Signal port t
  busesQueueAtStop : FIFOQueue
  getIDBusLeave : GetAttribute  AttributeName=ID  EvaluatedDefaultAttributeValue={ []}
      settings: OutputPortMap=o1
  busOut : PMIOPort  Port=1  Side=Right
  busIn : PMIOPort  Port=2  Side=Left
  idBusLeave : Outport
  wires:
  getIDBusLeave/1 -> idBusLeave/1
  dwellTime/1 -> Set Attribute3/1
  Clock2/1 -> T2E4/1
  T2E4/1 -> Set Attribute3/2
  Get Attribute5/2 -> Subsystem2/2(tStartSrvPax)
  Get Attribute5/1 -> Subsystem2/1(dwellTime)
  Subsystem2/1(dwellTimeNew) -> Infinite Server/1
  connections:
  busIn/RConn1 -- busesQueueAtStop/LConn1
  getIDBusLeave/RConn1 -- busOut/RConn1
  busesQueueAtStop/RConn1 -- Set Attribute3/LConn1
  Infinite Server/RConn1 -- getIDBusLeave/LConn1
  Set Attribute3/RConn1 -- FIFO Queue3/LConn1
  FIFO Queue3/RConn1 -- Get Attribute5/LConn1
  Get Attribute5/RConn1 -- DummyServer/LConn1
  Infinite Server/LConn1 -- DummyServer/RConn1

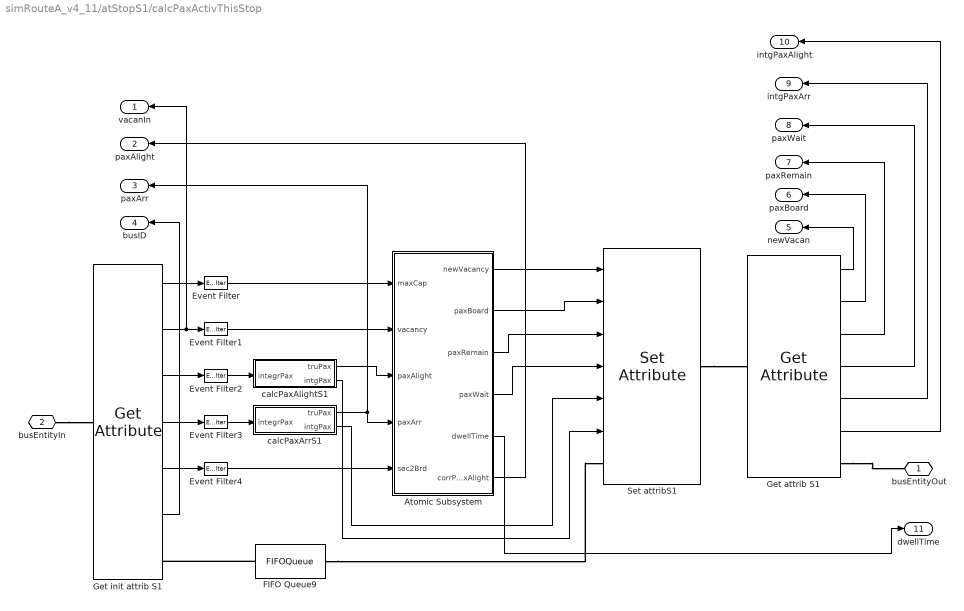
== system simRouteA_v4_11/atStopS1/calcPaxActivThisStop ==
  Atomic Subsystem : Subsystem  TreatAsAtomicUnit=on
  Event Filter{,1..4} (5 alike) : EventFilter  ExecuteSubsystem=Upon sample time hit  SignalEdgeType=Rising
  FIFO Queue9 : FIFOQueue
  Get attrib S1 : GetAttribute  AttributeName=vacancy|paxBoard|paxRemain|paxWait|intgPaxArr|intgPaxAlight  AttributeMissing=Error|Error|Error|Error|Error|Error  AttributeDefaultValue=1|1|1|1|1|1  AttributeTreatAsVector=1|1|1|1|1|1  AttributeSendTiming=After entity departure|After entity departure|After entity departure|After entity departure|After entity departure|After entity departure  EvaluatedDefaultAttributeValue={ []; []; []; []; []; []}
      settings: OutputPortMap=o1,o2,o3,o4,o5,o6
  Get init attrib S1 : GetAttribute  AttributeName=maxCap|vacancy|paxAlight|paxArr|sec2Brd|ID  AttributeMissing=Error|Error|Error|Error|Error|Error  AttributeDefaultValue=1|1|1|1|1|1  AttributeTreatAsVector=1|1|1|1|1|1  AttributeSendTiming=After entity departure|After entity departure|After entity departure|After entity departure|After entity departure|After entity departure  EvaluatedDefaultAttributeValue={ []; []; []; []; []; []}
      settings: OutputPortMap=o1,o2,o3,o4,o5,o6
  Set attribS1 : SetAttribute  AttributeName=vacancy|paxBoard|paxRemain|paxWait|intgPaxArr|intgPaxAlight  AttributeFrom=Signal port|Signal port|Signal port|Signal port|Signal port|Signal port  AttributeValue=1|1|1|1|1|1  AttributeTreatAsVector=1|1|1|1|1|1  EvaluatedAttributeValue={ []; []; []; []; []; [] }
      settings: InputPortMap=u0,u1,u2,u3,u4,u5
  calcPaxAlightS1 : Subsystem  TreatAsAtomicUnit=on
  calcPaxArrS1 : Subsystem  TreatAsAtomicUnit=on
  busEntityOut : PMIOPort  Port=1  Side=Right
  busEntityIn : PMIOPort  Port=2  Side=Left
  vacanIn : Outport
  paxAlight : Outport  Port=2
  paxArr : Outport  Port=3
  busID : Outport  Port=4
  newVacan : Outport  Port=5
  paxBoard : Outport  Port=6
  paxRemain : Outport  Port=7
  paxWait : Outport  Port=8
  intgPaxArr : Outport  Port=9
  intgPaxAlight : Outport  Port=10
  dwellTime : Outport  Port=11
  wires:
  Event Filter3/1 -> calcPaxArrS1/1(integrPax)
  Event Filter2/1 -> calcPaxAlightS1/1(integrPax)
  Get init attrib S1/6 -> busID/1
  Get init attrib S1/2 -> vacanIn/1, Event Filter1/1
  Get attrib S1/2 -> paxBoard/1
  Atomic Subsystem/1(newVacancy) -> Set attribS1/1
  Get attrib S1/1 -> newVacan/1
  Get attrib S1/3 -> paxRemain/1
  Get attrib S1/4 -> paxWait/1
  Event Filter/1 -> Atomic Subsystem/1(maxCap)
  Get init attrib S1/5 -> Event Filter4/1
  Atomic Subsystem/5(dwellTime) -> dwellTime/1
  Event Filter1/1 -> Atomic Subsystem/2(vacancy)
  Get init attrib S1/1 -> Event Filter/1
  Event Filter4/1 -> Atomic Subsystem/5(sec2Brd)
  Atomic Subsystem/2(paxBoard) -> Set attribS1/2
  Atomic Subsystem/3(paxRemain) -> Set attribS1/3
  Atomic Subsystem/4(paxWait) -> Set attribS1/4
  Get init attrib S1/4 -> Event Filter3/1
  Get init attrib S1/3 -> Event Filter2/1
  calcPaxAlightS1/1(truPax) -> Atomic Subsystem/3(paxAlight)
  calcPaxArrS1/1(truPax) -> Atomic Subsystem/4(paxArr), paxArr/1
  calcPaxArrS1/2(intgPax) -> Set attribS1/5
  calcPaxAlightS1/2(intgPax) -> Set attribS1/6
  Get attrib S1/5 -> intgPaxArr/1
  Get attrib S1/6 -> intgPaxAlight/1
  Atomic Subsystem/6(corrPaxAlight) -> paxAlight/1
  connections:
  busEntityIn/RConn1 -- Get init attrib S1/LConn1
  FIFO Queue9/LConn1 -- Get init attrib S1/RConn1
  Set attribS1/RConn1 -- Get attrib S1/LConn1
  Get attrib S1/RConn1 -- busEntityOut/RConn1
  FIFO Queue9/RConn1 -- Set attribS1/LConn1

== system simRouteA_v4_11/atStopS1/integrPaxAlightS1 ==
  ratePax : Inport
  Atomic Subsystem1 : Subsystem  TreatAsAtomicUnit=on
  Round1 : Rounding  Operator=round
  T2E1 : TimedToEventSignal
  accPax : Outport
  wires:
  Round1/1 -> T2E1/1
  T2E1/1 -> Atomic Subsystem1/1(In1)
  ratePax/1 -> Round1/1
  Atomic Subsystem1/1(Out1) -> accPax/1

== system simRouteA_v4_11/atStopS1/integrPaxArrS1 ==
  ratePax : Inport
  Atomic Subsystem1 : Subsystem  TreatAsAtomicUnit=on
  Round1 : Rounding  Operator=round
  T2E1 : TimedToEventSignal
  accPax : Outport
  wires:
  Round1/1 -> T2E1/1
  T2E1/1 -> Atomic Subsystem1/1(In1)
  ratePax/1 -> Round1/1
  Atomic Subsystem1/1(Out1) -> accPax/1

== system simRouteA_v4_11/atStopS10/busDwellThisStop ==
  dwellTime : Inport
  Clock2 : Clock
  DummyServer : SingleServer  ServiceTime=0
  FIFO Queue3 : FIFOQueue
  Get Attribute5 : GetAttribute  AttributeName=dwellTime|tStartSrvPax  AttributeMissing=Error|Error  AttributeDefaultValue=1|1  AttributeTreatAsVector=1|1  AttributeSendTiming=After entity departure|After entity departure  EvaluatedDefaultAttributeValue={ []; []}
      settings: OutputPortMap=o1,o2
  Infinite Server : InfiniteServer  ServiceTimeFrom=Signal port t
  Set Attribute3 : SetAttribute  AttributeName=dwellTime|tStartSrvPax  AttributeFrom=Signal port|Signal port  AttributeValue=1|1  AttributeTreatAsVector=1|1  EvaluatedAttributeValue={ []; [] }
      settings: InputPortMap=u0,u1
  Subsystem2 : Subsystem  TreatAsAtomicUnit=on
  T2E4 : TimedToEventSignal
  busWaitAtStop : SingleServer  Commented=on  ServiceTimeFrom=Signal port t
  busesQueueAtStop : FIFOQueue
  getIDBusLeave : GetAttribute  AttributeName=ID  EvaluatedDefaultAttributeValue={ []}
      settings: OutputPortMap=o1
  busOut : PMIOPort  Port=1  Side=Right
  busIn : PMIOPort  Port=2  Side=Left
  idBusLeave : Outport
  wires:
  getIDBusLeave/1 -> idBusLeave/1
  dwellTime/1 -> Set Attribute3/1
  Clock2/1 -> T2E4/1
  T2E4/1 -> Set Attribute3/2
  Get Attribute5/2 -> Subsystem2/2(tStartSrvPax)
  Get Attribute5/1 -> Subsystem2/1(dwellTime)
  Subsystem2/1(dwellTimeNew) -> Infinite Server/1
  connections:
  busIn/RConn1 -- busesQueueAtStop/LConn1
  getIDBusLeave/RConn1 -- busOut/RConn1
  busesQueueAtStop/RConn1 -- Set Attribute3/LConn1
  Infinite Server/RConn1 -- getIDBusLeave/LConn1
  Set Attribute3/RConn1 -- FIFO Queue3/LConn1
  FIFO Queue3/RConn1 -- Get Attribute5/LConn1
  Get Attribute5/RConn1 -- DummyServer/LConn1
  Infinite Server/LConn1 -- DummyServer/RConn1

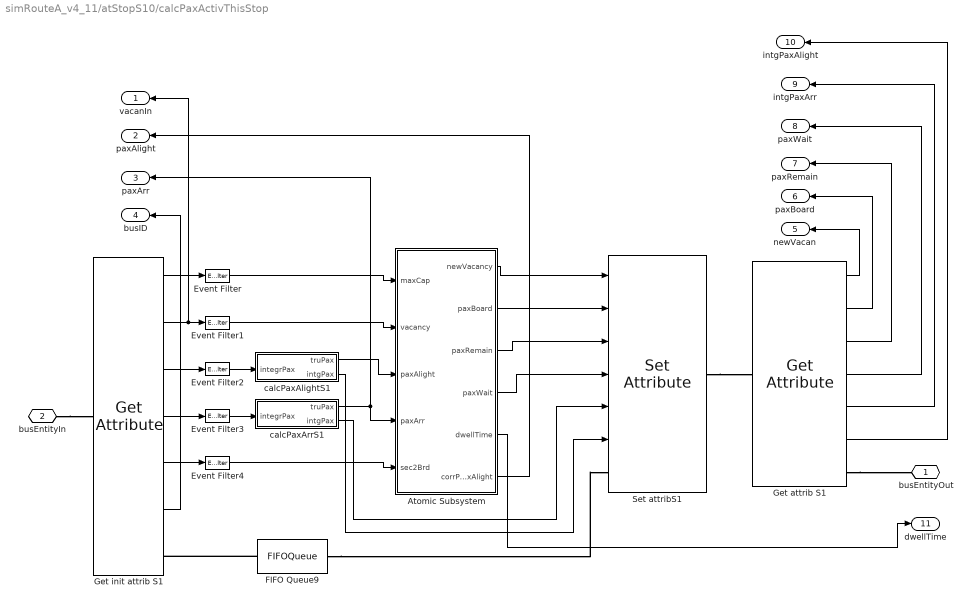
== system simRouteA_v4_11/atStopS10/calcPaxActivThisStop ==
  Atomic Subsystem : Subsystem  TreatAsAtomicUnit=on
  Event Filter{,1..4} (5 alike) : EventFilter  ExecuteSubsystem=Upon sample time hit  SignalEdgeType=Rising
  FIFO Queue9 : FIFOQueue
  Get attrib S1 : GetAttribute  AttributeName=vacancy|paxBoard|paxRemain|paxWait|intgPaxArr|intgPaxAlight  AttributeMissing=Error|Error|Error|Error|Error|Error  AttributeDefaultValue=1|1|1|1|1|1  AttributeTreatAsVector=1|1|1|1|1|1  AttributeSendTiming=After entity departure|After entity departure|After entity departure|After entity departure|After entity departure|After entity departure  EvaluatedDefaultAttributeValue={ []; []; []; []; []; []}
      settings: OutputPortMap=o1,o2,o3,o4,o5,o6
  Get init attrib S1 : GetAttribute  AttributeName=maxCap|vacancy|paxAlight|paxArr|sec2Brd|ID  AttributeMissing=Error|Error|Error|Error|Error|Error  AttributeDefaultValue=1|1|1|1|1|1  AttributeTreatAsVector=1|1|1|1|1|1  AttributeSendTiming=After entity departure|After entity departure|After entity departure|After entity departure|After entity departure|After entity departure  EvaluatedDefaultAttributeValue={ []; []; []; []; []; []}
      settings: OutputPortMap=o1,o2,o3,o4,o5,o6
  Set attribS1 : SetAttribute  AttributeName=vacancy|paxBoard|paxRemain|paxWait|intgPaxArr|intgPaxAlight  AttributeFrom=Signal port|Signal port|Signal port|Signal port|Signal port|Signal port  AttributeValue=1|1|1|1|1|1  AttributeTreatAsVector=1|1|1|1|1|1  EvaluatedAttributeValue={ []; []; []; []; []; [] }
      settings: InputPortMap=u0,u1,u2,u3,u4,u5
  calcPaxAlightS1 : Subsystem  TreatAsAtomicUnit=on
  calcPaxArrS1 : Subsystem  TreatAsAtomicUnit=on
  busEntityOut : PMIOPort  Port=1  Side=Right
  busEntityIn : PMIOPort  Port=2  Side=Left
  vacanIn : Outport
  paxAlight : Outport  Port=2
  paxArr : Outport  Port=3
  busID : Outport  Port=4
  newVacan : Outport  Port=5
  paxBoard : Outport  Port=6
  paxRemain : Outport  Port=7
  paxWait : Outport  Port=8
  intgPaxArr : Outport  Port=9
  intgPaxAlight : Outport  Port=10
  dwellTime : Outport  Port=11
  wires:
  Event Filter3/1 -> calcPaxArrS1/1(integrPax)
  Event Filter2/1 -> calcPaxAlightS1/1(integrPax)
  Get init attrib S1/6 -> busID/1
  Get init attrib S1/2 -> vacanIn/1, Event Filter1/1
  Get attrib S1/2 -> paxBoard/1
  Atomic Subsystem/1(newVacancy) -> Set attribS1/1
  Get attrib S1/1 -> newVacan/1
  Get attrib S1/3 -> paxRemain/1
  Get attrib S1/4 -> paxWait/1
  Event Filter/1 -> Atomic Subsystem/1(maxCap)
  Get init attrib S1/5 -> Event Filter4/1
  Atomic Subsystem/5(dwellTime) -> dwellTime/1
  Event Filter1/1 -> Atomic Subsystem/2(vacancy)
  Get init attrib S1/1 -> Event Filter/1
  Event Filter4/1 -> Atomic Subsystem/5(sec2Brd)
  Atomic Subsystem/2(paxBoard) -> Set attribS1/2
  Atomic Subsystem/3(paxRemain) -> Set attribS1/3
  Atomic Subsystem/4(paxWait) -> Set attribS1/4
  Get init attrib S1/4 -> Event Filter3/1
  Get init attrib S1/3 -> Event Filter2/1
  calcPaxAlightS1/1(truPax) -> Atomic Subsystem/3(paxAlight)
  calcPaxArrS1/1(truPax) -> Atomic Subsystem/4(paxArr), paxArr/1
  calcPaxArrS1/2(intgPax) -> Set attribS1/5
  calcPaxAlightS1/2(intgPax) -> Set attribS1/6
  Get attrib S1/5 -> intgPaxArr/1
  Get attrib S1/6 -> intgPaxAlight/1
  Atomic Subsystem/6(corrPaxAlight) -> paxAlight/1
  connections:
  busEntityIn/RConn1 -- Get init attrib S1/LConn1
  FIFO Queue9/LConn1 -- Get init attrib S1/RConn1
  Set attribS1/RConn1 -- Get attrib S1/LConn1
  Get attrib S1/RConn1 -- busEntityOut/RConn1
  FIFO Queue9/RConn1 -- Set attribS1/LConn1

== system simRouteA_v4_11/atStopS10/integrPaxAlightS1 ==
  ratePax : Inport
  Atomic Subsystem1 : Subsystem  TreatAsAtomicUnit=on
  Round1 : Rounding  Operator=round
  T2E1 : TimedToEventSignal
  accPax : Outport
  wires:
  Round1/1 -> T2E1/1
  T2E1/1 -> Atomic Subsystem1/1(In1)
  ratePax/1 -> Round1/1
  Atomic Subsystem1/1(Out1) -> accPax/1

== system simRouteA_v4_11/atStopS10/integrPaxArrS1 ==
  ratePax : Inport
  Atomic Subsystem1 : Subsystem  TreatAsAtomicUnit=on
  Round1 : Rounding  Operator=round
  T2E1 : TimedToEventSignal
  accPax : Outport
  wires:
  Round1/1 -> T2E1/1
  T2E1/1 -> Atomic Subsystem1/1(In1)
  ratePax/1 -> Round1/1
  Atomic Subsystem1/1(Out1) -> accPax/1

== system simRouteA_v4_11/atStopS11/busDwellThisStop ==
  dwellTime : Inport
  Clock2 : Clock
  DummyServer : SingleServer  ServiceTime=0
  FIFO Queue3 : FIFOQueue
  Get Attribute5 : GetAttribute  AttributeName=dwellTime|tStartSrvPax  AttributeMissing=Error|Error  AttributeDefaultValue=1|1  AttributeTreatAsVector=1|1  AttributeSendTiming=After entity departure|After entity departure  EvaluatedDefaultAttributeValue={ []; []}
      settings: OutputPortMap=o1,o2
  Infinite Server : InfiniteServer  ServiceTimeFrom=Signal port t
  Set Attribute3 : SetAttribute  AttributeName=dwellTime|tStartSrvPax  AttributeFrom=Signal port|Signal port  AttributeValue=1|1  AttributeTreatAsVector=1|1  EvaluatedAttributeValue={ []; [] }
      settings: InputPortMap=u0,u1
  Subsystem2 : Subsystem  TreatAsAtomicUnit=on
  T2E4 : TimedToEventSignal
  busWaitAtStop : SingleServer  Commented=on  ServiceTimeFrom=Signal port t
  busesQueueAtStop : FIFOQueue
  getIDBusLeave : GetAttribute  AttributeName=ID  EvaluatedDefaultAttributeValue={ []}
      settings: OutputPortMap=o1
  busOut : PMIOPort  Port=1  Side=Right
  busIn : PMIOPort  Port=2  Side=Left
  idBusLeave : Outport
  wires:
  getIDBusLeave/1 -> idBusLeave/1
  dwellTime/1 -> Set Attribute3/1
  Clock2/1 -> T2E4/1
  T2E4/1 -> Set Attribute3/2
  Get Attribute5/2 -> Subsystem2/2(tStartSrvPax)
  Get Attribute5/1 -> Subsystem2/1(dwellTime)
  Subsystem2/1(dwellTimeNew) -> Infinite Server/1
  connections:
  busIn/RConn1 -- busesQueueAtStop/LConn1
  getIDBusLeave/RConn1 -- busOut/RConn1
  busesQueueAtStop/RConn1 -- Set Attribute3/LConn1
  Infinite Server/RConn1 -- getIDBusLeave/LConn1
  Set Attribute3/RConn1 -- FIFO Queue3/LConn1
  FIFO Queue3/RConn1 -- Get Attribute5/LConn1
  Get Attribute5/RConn1 -- DummyServer/LConn1
  Infinite Server/LConn1 -- DummyServer/RConn1
